simulink model "s12_euler_hllc_flux_ref"  (R2026a)
settings: Solver=FixedStepDiscrete  StopTime=0
model workspace (MAT data in the model file):
  S12_HLLC_Gamma = Simulink.Parameter
  S12_HLLC_Gamma.Value = 1.4
  S12_HLLC_Gamma.Complexity = 'real'
  S12_HLLC_Gamma.Dimensions = [1 1]
  S12_HLLC_Gamma.Description = 'Heat capacity ratio'
  S12_HLLC_Gamma.DataType = 'auto'
  S12_HLLC_Gamma.DocUnits = '1'
  S12_HLLC_PL = Simulink.Parameter
  S12_HLLC_PL.Value = 100000
  S12_HLLC_PL.Complexity = 'real'
  S12_HLLC_PL.Dimensions = [1 1]
  S12_HLLC_PL.Description = 'Left pressure'
  S12_HLLC_PL.DataType = 'auto'
  S12_HLLC_PL.DocUnits = 'Pa'
  S12_HLLC_PR = Simulink.Parameter
  S12_HLLC_PR.Value = 10000
  S12_HLLC_PR.Complexity = 'real'
  S12_HLLC_PR.Dimensions = [1 1]
  S12_HLLC_PR.Description = 'Right pressure'
  S12_HLLC_PR.DataType = 'auto'
  S12_HLLC_PR.DocUnits = 'Pa'
  S12_HLLC_RhoL = Simulink.Parameter
  S12_HLLC_RhoL.Value = 1
  S12_HLLC_RhoL.Complexity = 'real'
  S12_HLLC_RhoL.Dimensions = [1 1]
  S12_HLLC_RhoL.Description = 'Left density'
  S12_HLLC_RhoL.DataType = 'auto'
  S12_HLLC_RhoL.DocUnits = 'kg/m^3'
  S12_HLLC_RhoR = Simulink.Parameter
  S12_HLLC_RhoR.Value = 0.125
  S12_HLLC_RhoR.Complexity = 'real'
  S12_HLLC_RhoR.Dimensions = [1 1]
  S12_HLLC_RhoR.Description = 'Right density'
  S12_HLLC_RhoR.DataType = 'auto'
  S12_HLLC_RhoR.DocUnits = 'kg/m^3'
  S12_HLLC_UL = Simulink.Parameter
  S12_HLLC_UL.Value = 0
  S12_HLLC_UL.Complexity = 'real'
  S12_HLLC_UL.Dimensions = [1 1]
  S12_HLLC_UL.Description = 'Left velocity'
  S12_HLLC_UL.DataType = 'auto'
  S12_HLLC_UL.DocUnits = 'm/s'
  S12_HLLC_UR = Simulink.Parameter
  S12_HLLC_UR.Value = 0
  S12_HLLC_UR.Complexity = 'real'
  S12_HLLC_UR.Dimensions = [1 1]
  S12_HLLC_UR.Description = 'Right velocity'
  S12_HLLC_UR.DataType = 'auto'
  S12_HLLC_UR.DocUnits = 'm/s'
settings Model: Creator=Jovi  LastModifiedBy=Jovi

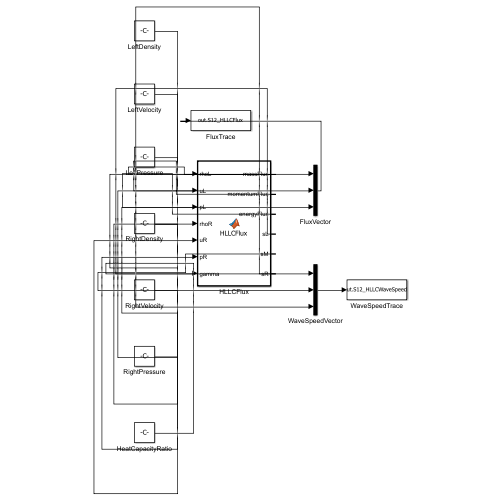
[thumbnail: Simulink's stored preview of the top-level diagram]
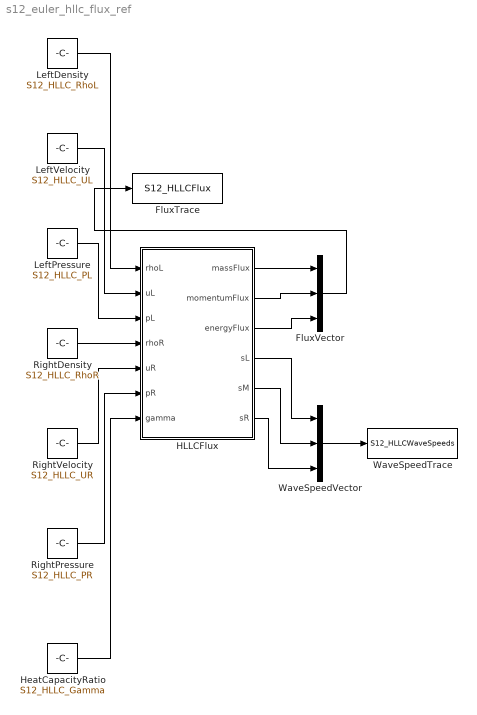
== system s12_euler_hllc_flux_ref ==
  FluxTrace : ToWorkspace  VariableName=S12_HLLCFlux
      settings: MaxDataPoints=100
  FluxVector : Mux  Inputs=3
  HLLCFlux : MATLAB Function  TreatAsAtomicUnit=on
  HeatCapacityRatio : Constant  Value=S12_HLLC_Gamma
  LeftDensity : Constant  Value=S12_HLLC_RhoL
  LeftPressure : Constant  Value=S12_HLLC_PL
  LeftVelocity : Constant  Value=S12_HLLC_UL
  RightDensity : Constant  Value=S12_HLLC_RhoR
  RightPressure : Constant  Value=S12_HLLC_PR
  RightVelocity : Constant  Value=S12_HLLC_UR
  WaveSpeedTrace : ToWorkspace  VariableName=S12_HLLCWaveSpeeds
      settings: MaxDataPoints=100
  WaveSpeedVector : Mux  Inputs=3
  wires:
  WaveSpeedVector/1 -> WaveSpeedTrace/1
  FluxVector/1 -> FluxTrace/1
  LeftDensity/1 -> HLLCFlux/1(rhoL)
  LeftVelocity/1 -> HLLCFlux/2(uL)
  LeftPressure/1 -> HLLCFlux/3(pL)
  RightDensity/1 -> HLLCFlux/4(rhoR)
  RightVelocity/1 -> HLLCFlux/5(uR)
  RightPressure/1 -> HLLCFlux/6(pR)
  HeatCapacityRatio/1 -> HLLCFlux/7(gamma)
  HLLCFlux/1(massFlux) -> FluxVector/1
  HLLCFlux/2(momentumFlux) -> FluxVector/2
  HLLCFlux/3(energyFlux) -> FluxVector/3
  HLLCFlux/4(sL) -> WaveSpeedVector/1
  HLLCFlux/5(sM) -> WaveSpeedVector/2
  HLLCFlux/6(sR) -> WaveSpeedVector/3

== matlab function s12_euler_hllc_flux_ref/HLLCFlux ==
  data: rhoL input; massFlux output; uL input; pL input; rhoR input; uR input; pR input; gamma input; momentumFlux output; energyFlux output; sL output; sM output; sR output
function [massFlux,momentumFlux,energyFlux,sL,sM,sR] = HLLCFlux(rhoL,uL,pL,rhoR,uR,pR,gamma)
%#codegen
energyL = pL/(gamma-1) + 0.5*rhoL*uL*uL;
energyR = pR/(gamma-1) + 0.5*rhoR*uR*uR;
soundL = sqrt(gamma*pL/rhoL);
soundR = sqrt(gamma*pR/rhoR);
sL = min(uL-soundL,uR-soundR);
sR = max(uL+soundL,uR+soundR);
denominator = rhoL*(sL-uL) - rhoR*(sR-uR);
sM = (pR-pL + rhoL*uL*(sL-uL) - rhoR*uR*(sR-uR))/denominator;
fluxL = [rhoL*uL; rhoL*uL*uL+pL; uL*(energyL+pL)];
fluxR = [rhoR*uR; rhoR*uR*uR+pR; uR*(energyR+pR)];
stateL = [rhoL; rhoL*uL; energyL];
stateR = [rhoR; rhoR*uR; energyR];
if sL >= 0
    flux = fluxL;
elseif sM >= 0
    rhoStarL = rhoL*(sL-uL)/(sL-sM);
    energyStarL = rhoStarL*(energyL/rhoL + (sM-uL)*(sM + pL/(rhoL*(sL-uL))));
    stateStarL = [rhoStarL; rhoStarL*sM; energyStarL];
    flux = fluxL + sL*(stateStarL-stateL);
elseif sR > 0
    rhoStarR = rhoR*(sR-uR)/(sR-sM);
    energyStarR = rhoStarR*(energyR/rhoR + (sM-uR)*(sM + pR/(rhoR*(sR-uR))));
    stateStarR = [rhoStarR; rhoStarR*sM; energyStarR];
    flux = fluxR + sR*(stateStarR-stateR);
else
    flux = fluxR;
end
massFlux = flux(1);
momentumFlux = flux(2);
energyFlux = flux(3);
end
